simulink model "state_feedback"  (R2019a)
settings: Solver=VariableStepAuto  StartTime=0.0  StopTime=10  RelTol=1e-3
settings Model: Creator=harkib  LastModifiedBy=harki
settings DataIOCC: ReturnWorkspaceOutputs=off
settings DebuggingCC: PregeneratedLibrarySubsystemCodeDiagnostic=none  ArithmeticOperatorsInVariantConditions=warning
settings SFSimCC: SimUseLocalCustomCode=off
settings RTWCC: RTWUseLocalCustomCode=off

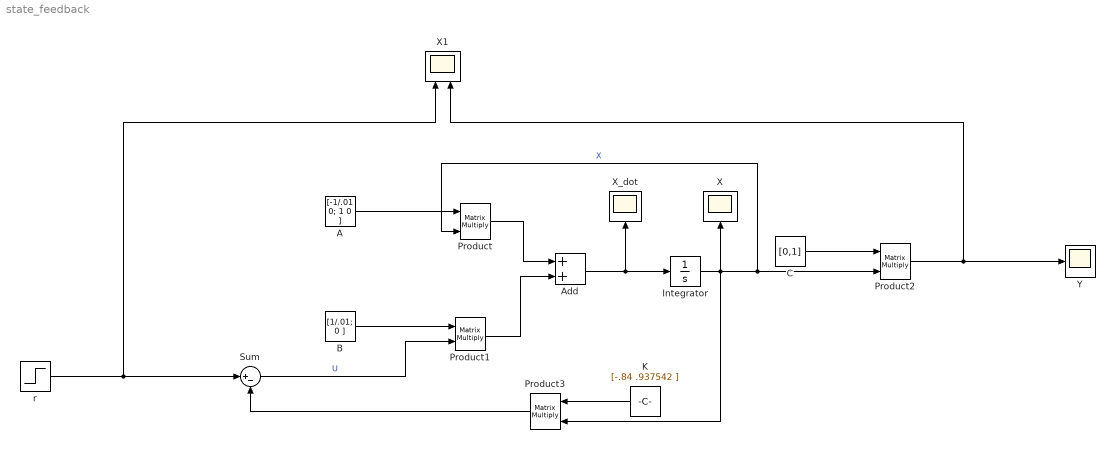
== system state_feedback ==
  A : Constant  Value=[-1/.01 0; 1 0 ]  VectorParams1D=off
  Add : Sum
  B : Constant  Value=[1/.01; 0 ]  VectorParams1D=off
  C : Constant  Value=[0,1]  VectorParams1D=off
  Integrator : Integrator
  K : Constant  Value=[-.84 .937542 ]  VectorParams1D=off
  Product{,1..3} (4 alike) : Product  Multiplication=Matrix(*)
  Sum : Sum  Inputs=|+-
  X : Scope
  X1 : Scope  NumInputPorts=2
  X_dot : Scope
  Y : Scope
  r : Step  SampleTime=0
  wires:
  Add/1 -> X_dot/1, Integrator/1
  Product1/1 -> Add/2
  Product/1 -> Add/1
  B/1 -> Product1/1
  A/1 -> Product/1
  r/1 -> X1/1, Sum/1
  K/1 -> Product3/1
  Integrator/1 -> Product3/2, Product2/2, Product/2, X/1  "X"
  Product3/1 -> Sum/2
  Sum/1 -> Product1/2  "U"
  C/1 -> Product2/1
  Product2/1 -> X1/2, Y/1
